simulink model "HybridPowertrain_TestBench_Final"  (R2017a)
settings: Solver=ode1  StartTime=0.0  StopTime=1400  FixedStep=0.01  RelTol=1e-3  EnableMultiTasking=on
undefined symbols (not defined in the file): AccActPos, air, Atm_temp, bms_inletair_temp, BMS_IstStrom, bms_maxchargecurrent, bms_maxdischargecurrent, BMS_Notfallkuehlung, BMS_SOC, BrkPdlPos, cal, Cells, Chg, D1_Commanded_Torque, D1_DC_Bus_Voltage, D2_Motor_Speed, D2_Torque_Feedback, DriverControls, EcoCAR3_Lib, Em, EngActStdyStTorq, Engine, EngSpd, env, ESS, fd, g, gb, Gearbox, GearBox, gps_lat, gps_long, Grade, I_loss, IMG, InstFuelConsmpRate, KeyPosition, lib_ESS_plant_V1_2, Loss, max_vehicle_rad_air_flow, mot, mph2kph, mph2ms, NeutralGear, ParkGear, PPEI_Engine_General_Status_2__ThrPos, PTEI_Engine_Torque_Status__EngActStdyStTorq, R_0, R_1, Ratio, RegenBrkDisable, rho, SampleTime, ShiftLeverPosition, SOC_bp, SOC_init, Spd, Speed, SW_CS_ON, SW_Engine_ON ... (+15)
libraries: simulink x39, fl_lib x13, nesl_utility x8, Utility x1, EC2_libraries x1
(part 5 of 5)

== system HybridPowertrain_TestBench_Final/IMG/Soft MCU/Torque Calculation/max torque /Divide by zero ==
  In1 : Inport
  Compare To Constant : simulink/Logic and Bit Operations/Compare To Constant  relop=<=  const=3.0  OutDataTypeStr=boolean
  Constant1 : Constant
  Switch2 : Switch  Criteria=u2 > Threshold
  Out1 : Outport
  wires:
  Constant1/1 -> Switch2/1
  Compare To Constant/1 -> Switch2/2
  In1/1 -> Switch2/3, Compare To Constant/1
  Switch2/1 -> Out1/1

== system HybridPowertrain_TestBench_Final/IMG/Soft MCU/Torque Calculation/max torque /Heat index ==
  note: Heat index calculation
  cont torque : Inport
  torque : Inport  Port=2
  Abs : Abs  SaturateOnIntegerOverflow=on
  Divide : Subsystem  mask(Divide){}
      mask Display: disp('Divide')
  Heat Energy Factor : Integrator  InitialCondition=-0.3  LimitOutput=on  UpperSaturationLimit=1  LowerSaturationLimit=-0.3
  Heating Constant : Gain  Gain=0.3/mot.plant.init.t_max_trq  SaturateOnIntegerOverflow=on  OutDataTypeStr=Inherit: Same as input  ParamDataTypeStr=Inherit: Same as input
  Saturation : Saturate  UpperLimit=1  LowerLimit=0
  Sum : Sum  Inputs=+-  SaturateOnIntegerOverflow=on  InputSameDT=on  OutDataTypeStr=Inherit: Same as first input
  motor inertia (Nms^2\rad)5 : Constant
  Heat index : Outport
  wires:
  cont torque/1 -> Divide/2(denominator)
  Abs/1 -> Sum/1
  Saturation/1 -> Heat index/1
  motor inertia (Nms^2\rad)5/1 -> Sum/2
  Divide/1(quotient) -> Abs/1
  Sum/1 -> Heating Constant/1
  Heating Constant/1 -> Heat Energy Factor/1
  Heat Energy Factor/1 -> Saturation/1
  torque/1 -> Divide/1(numerator)

== system HybridPowertrain_TestBench_Final/Transmission/Transmission Plant/Gearbox/Speed Calculation/P//N ==
  torque input : Inport
  Inertia Input : Inport  Port=2
  gear : Inport  Port=3
  inital speed : Inport  Port=4
  (0,inf) : Saturate  UpperLimit=1100  LowerLimit=0
  Add : Sum
  Bus Selector : BusSelector  Commented=on  OutputSignals=drv_BPP_req_[%]
  Compare To Constant : simulink/Logic and Bit Operations/Compare To Constant  Commented=on  relop=<=  const=1  OutDataTypeStr=boolean
  Compare To Constant1 : simulink/Logic and Bit Operations/Compare To Constant  Commented=on  relop=>  const=2  OutDataTypeStr=boolean
  Compare To Constant2 : simulink/Logic and Bit Operations/Compare To Constant  Commented=on  relop=<=  const=1000  OutDataTypeStr=boolean
  Fcn2 : Fcn  Expr=u==0
  From10 : From  Commented=on  GotoTag=Driver_Request  TagVisibility=global
  Inertias : Constant  Value=Gearbox.InputShaftInertia
  Integrator : Integrator  ExternalReset=rising  InitialConditionSource=external
  Logical Operator : Logic  Commented=on  Inputs=3  AllPortsSameDT=off  OutDataTypeStr=boolean
  Logical Operator1 : Logic  Operator=OR  AllPortsSameDT=off  OutDataTypeStr=boolean
  Memory : Memory
  Subsystem2 : Subsystem
      mask Display: disp('divider')
  Sum : Sum  Inputs=-+|  SaturateOnIntegerOverflow=on  InputSameDT=on  OutDataTypeStr=Inherit: Same as first input
  Switch : Switch  Commented=on  Criteria=u2 > Threshold
  input shaft free wheeling losses : Subsystem
  speed : Outport
  decel : Outport  Port=2
  wires:
  Inertia Input/1 -> Add/1
  Fcn2/1 -> Logical Operator1/2
  Subsystem2/1(Out1) -> decel/1, Integrator/1
  Memory/1 -> Integrator/3
  (0,inf)/1 -> speed/1
  torque input/1 -> Sum/2
  Sum/1 -> Subsystem2/1(In1)
  input shaft free wheeling losses/1(input shaft decel) -> Sum/1
  Integrator/1 -> input shaft free wheeling losses/1(input shaft speed), Switch/1, (0,inf)/1
  gear/1 -> Fcn2/1, Compare To Constant/1
  Compare To Constant/1 -> Logical Operator/2
  Logical Operator/1 -> Logical Operator1/1, Switch/2
  From10/1 -> Bus Selector/1
  Bus Selector/1 -> Compare To Constant1/1  "<drv_BPP_req_[%]>"
  Compare To Constant1/1 -> Logical Operator/1
  Compare To Constant2/1 -> Logical Operator/3
  inital speed/1 -> Compare To Constant2/1, Memory/1
  Logical Operator1/1 -> Integrator/2
  Add/1 -> Subsystem2/2(In2)
  Inertias/1 -> Add/2

== system HybridPowertrain_TestBench_Final/Transmission/Transmission Plant/Gearbox/Speed Calculation/R//D ==
  spd in : Inport
  gear number : Inport  Port=2
  speed1 : Inport  Port=3
  Bus Selector : BusSelector  OutputSignals=drv_BPP_req_[%]
  Compare To Constant : simulink/Logic and Bit Operations/Compare To Constant  relop=<=  const=1  OutDataTypeStr=boolean
  Compare To Constant1 : simulink/Logic and Bit Operations/Compare To Constant  relop=>  const=0.4  OutDataTypeStr=boolean
  Compare To Constant2 : simulink/Logic and Bit Operations/Compare To Constant  relop=<=  const=1000  OutDataTypeStr=boolean
  Constant5 : Constant
  Constant6 : Constant  Value=gb.plant.init.shift_time
  Integrator : Integrator  ExternalReset=rising
  Logical Operator : Logic  Inputs=3  AllPortsSameDT=off  OutDataTypeStr=boolean
  Relational Operator4 : RelationalOperator  Operator=~=  RndMeth=Nearest  InputSameDT=on
  Relational Operator5 : RelationalOperator  Operator=<=  RndMeth=Nearest  InputSameDT=on
  S-R Flip-Flop : Subsystem  mask(SRFlipFlop){initial_condition=0}
      mask prompts: initial_condition "Initial condition:"
      mask help: S-R Flip Flop Block
  Switch : Switch  Threshold=0.5  SaturateOnIntegerOverflow=on  InputSameDT=on
  Switch1 : Switch  Criteria=u2 > Threshold
  Transfer Fcn : TransferFcn  Denominator=[.2 1]
  Unit Delay7 : Memory
  term2 : Terminator
  spd in filtered : Outport
  wires:
  spd in/1 -> Transfer Fcn/1, Switch/3, Switch1/3, Compare To Constant2/1
  Relational Operator5/1 -> S-R Flip-Flop/2(R)
  S-R Flip-Flop/1(Q) -> Switch/2
  Integrator/1 -> Relational Operator5/2
  Relational Operator4/1 -> S-R Flip-Flop/1(S), Integrator/2
  Unit Delay7/1 -> Relational Operator4/2
  S-R Flip-Flop/2(!Q) -> term2/1
  Constant6/1 -> Relational Operator5/1
  Constant5/1 -> Integrator/1
  gear number/1 -> Compare To Constant/1, Unit Delay7/1, Relational Operator4/1
  [Driver_Request2] -> Bus Selector/1
  Bus Selector/1 -> Compare To Constant1/1  "<drv_BPP_req_[%]>"
  Compare To Constant1/1 -> Logical Operator/1
  Compare To Constant/1 -> Logical Operator/2
  Logical Operator/1 -> Switch1/2
  Compare To Constant2/1 -> Logical Operator/3
  Switch1/1 -> spd in filtered/1
  speed1/1 -> Switch1/1
  Transfer Fcn/1 -> Switch/1

== system HybridPowertrain_TestBench_Final/Transmission/Transmission Plant/Gearbox/Subsystem1/Blending (state dependent) ==
  Input : Inport
  Control (state) : Inport  Port=2
  Linear spline : Fcn  Expr=(u<xl)*yl + (xl<=u)*(u<xc)*((yc-yl)*(u-xl)/(xc-xl)+yl) + (xc<=u)*(u<xr)*((yc-yr)*(u-xr)/(xc-xr)+yr) + (xr<=u)*yr
  Product2 : Product  SaturateOnIntegerOverflow=on  InputSameDT=on  OutDataTypeStr=Inherit: Same as first input
  Output : Outport
  wires:
  Control (state)/1 -> Linear spline/1
  Product2/1 -> Output/1
  Linear spline/1 -> Product2/2
  Input/1 -> Product2/1

== system HybridPowertrain_TestBench_Final/Transmission/Transmission Plant/Gearbox/Torque calculation/Blending (state dependent) ==
  Input : Inport
  Control (state) : Inport  Port=2
  Linear spline : Fcn  Expr=(u<xl)*yl + (xl<=u)*(u<xc)*((yc-yl)*(u-xl)/(xc-xl)+yl) + (xc<=u)*(u<xr)*((yc-yr)*(u-xr)/(xc-xr)+yr) + (xr<=u)*yr
  Product2 : Product  SaturateOnIntegerOverflow=on  InputSameDT=on  OutDataTypeStr=Inherit: Same as first input
  Output : Outport
  wires:
  Control (state)/1 -> Linear spline/1
  Product2/1 -> Output/1
  Linear spline/1 -> Product2/2
  Input/1 -> Product2/1

== system HybridPowertrain_TestBench_Final/ESS/Soft BMS/Limits/Average Current/60 sec rolling average1/1sec trigger ==
  0 : Constant  Value=0
  Compare To Constant : simulink/Logic and Bit Operations/Compare To Constant  relop=<=  const=3.0  OutDataTypeStr=boolean
  Data Type Conversion : DataTypeConversion
  Sum2 : Sum  Inputs=|++
  Switch : Switch  Threshold=0.5
  accumulate2 : Memory  InheritSampleTime=on
  tloop : Constant  Value=tloop
  Trigger : Outport
  wires:
  Data Type Conversion/1 -> Trigger/1, Switch/2
  0/1 -> Switch/1
  Compare To Constant/1 -> Data Type Conversion/1
  Switch/1 -> accumulate2/1
  Sum2/1 -> Switch/3, Compare To Constant/1
  accumulate2/1 -> Sum2/2
  tloop/1 -> Sum2/1

== system HybridPowertrain_TestBench_Final/ESS/Soft BMS/Limits/Average Current/60 sec rolling average1/60 sec average ==
  1sec : Inport
  Enable : EnablePort
  60 second : Delay  DelayLength=60  InputProcessing=Inherited  SampleTime=tloop
  Gain2 : Gain  Gain=1/60
  Sum2 : Sum  Inputs=++-
  accumulate2 : Memory  InheritSampleTime=on
  Average : Outport
  wires:
  1sec/1 -> Sum2/2, 60 second/1
  Gain2/1 -> Average/1
  accumulate2/1 -> Sum2/1
  60 second/1 -> Sum2/3
  Sum2/1 -> Gain2/1, accumulate2/1

== system HybridPowertrain_TestBench_Final/ESS/Soft BMS/Limits/Average Current/60 sec rolling average2/1sec trigger ==
  0 : Constant  Value=0
  Compare To Constant : simulink/Logic and Bit Operations/Compare To Constant  relop=<=  const=3.0  OutDataTypeStr=boolean
  Data Type Conversion : DataTypeConversion
  Sum2 : Sum  Inputs=|++
  Switch : Switch  Threshold=0.5
  accumulate2 : Memory  InheritSampleTime=on
  tloop : Constant  Value=tloop
  Trigger : Outport
  wires:
  Data Type Conversion/1 -> Trigger/1, Switch/2
  0/1 -> Switch/1
  Compare To Constant/1 -> Data Type Conversion/1
  Switch/1 -> accumulate2/1
  Sum2/1 -> Switch/3, Compare To Constant/1
  accumulate2/1 -> Sum2/2
  tloop/1 -> Sum2/1

== system HybridPowertrain_TestBench_Final/ESS/Soft BMS/Limits/Average Current/60 sec rolling average2/60 sec average ==
  1sec : Inport
  Enable : EnablePort
  60 second : Delay  DelayLength=60  InputProcessing=Inherited  SampleTime=tloop
  Gain2 : Gain  Gain=1/60
  Sum2 : Sum  Inputs=++-
  accumulate2 : Memory  InheritSampleTime=on
  Average : Outport
  wires:
  1sec/1 -> Sum2/2, 60 second/1
  Gain2/1 -> Average/1
  accumulate2/1 -> Sum2/1
  60 second/1 -> Sum2/3
  Sum2/1 -> Gain2/1, accumulate2/1

== system HybridPowertrain_TestBench_Final/IMG/Soft MCU/Torque Calculation/max torque /Heat index/Divide ==
  note: Take care of
      | division by 0
  numerator : Inport
  denominator : Inport  Port=2
  Fcn : Fcn  Expr=u[1] / ( u[2] + eps*(u[2]==0) )
  Mux : Mux  Inputs=2
  quotient : Outport
  wires:
  denominator/1 -> Mux/2
  Fcn/1 -> quotient/1
  numerator/1 -> Mux/1
  Mux/1 -> Fcn/1

== system HybridPowertrain_TestBench_Final/Transmission/Transmission Plant/Gearbox/Speed Calculation/P//N/Subsystem2 ==
  In1 : Inport
  In2 : Inport  Port=2
  Fcn : Fcn  Expr=u[1]/(u[2]+eps)*(u[2]!=0)
  Mux : Mux  Inputs=2
  Out1 : Outport
  wires:
  Mux/1 -> Fcn/1
  In1/1 -> Mux/1
  Fcn/1 -> Out1/1
  In2/1 -> Mux/2

== system HybridPowertrain_TestBench_Final/Transmission/Transmission Plant/Gearbox/Speed Calculation/P//N/input shaft free wheeling losses ==
  input shaft speed : Inport
  Constant1 : Constant  Value=0
  Fcn1 : Fcn  Expr=u==0
  Gain1 : Gain  Gain=0.15  SaturateOnIntegerOverflow=on  OutDataTypeStr=Inherit: Same as input  ParamDataTypeStr=Inherit: Same as input
  Switch2 : Switch  Threshold=0.5  SaturateOnIntegerOverflow=on  InputSameDT=on
  input shaft decel : Outport
  wires:
  input shaft speed/1 -> Switch2/3, Fcn1/1
  Fcn1/1 -> Switch2/2
  Gain1/1 -> input shaft decel/1
  Switch2/1 -> Gain1/1
  Constant1/1 -> Switch2/1

== system HybridPowertrain_TestBench_Final/Transmission/Transmission Plant/Gearbox/Speed Calculation/R//D/S-R Flip-Flop ==
  S : Inport
  R : Inport  Port=2
  Demux : Demux  Outputs=2
  Logic : CombinatorialLogic  TruthTable=[0 1;0 1;1 0;0 1;1 0;0 1;1 0;1 0]
  Memory : Memory  X0=initial_condition  InheritSampleTime=on
  Mux : Mux  Inputs=3
  Q : Outport  InitialOutput=0
  !Q : Outport  Port=2  InitialOutput=1
  wires:
  R/1 -> Mux/3
  S/1 -> Mux/2
  Memory/1 -> Mux/1
  Demux/1 -> Memory/1, Q/1
  Demux/2 -> !Q/1
  Logic/1 -> Demux/1
  Mux/1 -> Logic/1

== stateflow chart HybridPowertrain_TestBench_Final/ESS/Soft BMS/RollingAliveCnt1/Rolling Alive Counter ==
  state RollingAliveCounter
    state Count1
      en: RollingAliveCnt = 0;
    state Count2
      en: RollingAliveCnt = 1;
    state Count3
      en: RollingAliveCnt = 2;
    state Count4
      en: RollingAliveCnt = 3;
    (default) -> Count1
    Count4 -> Count1 : after(0.01,sec)
    Count1 -> Count2 : after(0.01,sec)
    Count2 -> Count3 : after(0.01,sec)
    Count3 -> Count4 : after(0.01,sec)
  data: RollingAliveCnt output int8 =0

== stateflow chart HybridPowertrain_TestBench_Final/ESS/Soft BMS/State Machine1/Startup_Shutdown_EPO_Sequence ==
  state BCM_ON
    state Default_Error_State
      en: BMS_Init_abgeschlossen=1;
      BMS_IstModus=5;
    state Standby
      en: BMS_Init_abgeschlossen=1;
      BMS_IstModus=0;
    state Normal_Driving
      en: NHM_BMS_Car_WakeUp=1;
      BMS_IstModus=1;
      BMS_Init_abgeschlossen=1;
      during: timer++;
    state Charging
      en:BMS_IstModus=4;
      BMS_Init_abgeschlossen =1;
      during: timer++;
    (default) -> Default_Error_State : [T_15&&T_30]
    Charging -> Default_Error_State [order 1] : [!T_30C]
    Normal_Driving -> Default_Error_State [order 1] : [!T_30C]
    (junction 134) -> Default_Error_State [order 2] : after(15, sec)[!T_30C]
    Default_Error_State -> Standby : [MO_BMS_Sollmodus==0&&...
        | Diag_Rq_Fktnl_Data_OBD==1]
        | %ErrorClear
    (junction 134) -> Standby [order 1] : [T_30C]
    Standby -> (junction 134) [order 3] : [!T_30C]
    Standby -> Charging [order 1] : [T_30C&&MO_BMS_Sollmodus==4]
        | %Standby>Charging
    Standby -> Normal_Driving [order 2] : [T_30C&&MO_BMS_Sollmodus==1]
        | {timer=0;}
        | %Standby>NormalDriving
    Normal_Driving -> Standby [order 2] : [T_30C&&MO_BMS_Sollmodus==0]
        | %NormalDriving>Standby
    Charging -> Standby [order 2] : [T_30C&&MO_BMS_Sollmodus==0]
        | %Charging>Standby
    Normal_Driving -> Charging [order 3] : [T_30C&&MO_BMS_Sollmodus==4] %NormalDriving>Charging
    Charging -> Normal_Driving [order 3] : [T_30C&&MO_BMS_Sollmodus==1] %Charging>NormalDriving
  state BCM_OFF
    state Prepare_to_Sleep
      en: NMH_BMS_Start_2=0;
      BMS_IstModus=5;
    state Ready_to_Sleep
      en: NMH_BMS_Normal_Mode_2=0;
      BMS_SleepInd=1;
      BMS_IstModus=5;
    state Bus_Sleep
      en: NMH_BMS_Start_1=0;
      BMS_SleepInd=1;
      BMS_IstModus=5;
    (default) -> Prepare_to_Sleep
    Prepare_to_Sleep -> Ready_to_Sleep : [timer>=0.05/tloop]
    Ready_to_Sleep -> Bus_Sleep : [timer>=0.05/tloop]
  note: !(veh_wake||chga_wake) || ...
      | !hsc_bcm_enable && !bcm_mainc_stat && bcm_cpwr_cmd]
  state EPO1
    BMS_Fehler_HS_offen=1;
    BMS_Fehler_HS_verschweisst =1;
    BMS_Fehler_HVBatt_Abschaltung=1;
    BMS_Fehler_HVBatt_Abschaltung_Anf=1;
    BMS_IstModus=5;
  state EPO
    BMS_Fehler_Notabschaltung_Crash=1;
    BMS_Fehler_Notabschaltung_Pilot=1;
    BMS_Fehler_Pilot=1;
    BMS_IstModus=5;
  (default) -> BCM_OFF
  BCM_OFF -> BCM_ON : [T_15&&T_30]
  BCM_ON -> BCM_OFF [order 1] : [T_15==0&&T_30==0]
  BCM_ON -> EPO1 [order 2] : [BattError]
  EPO1 -> BCM_OFF : [T_15==0&&T_30==0]
  EPO -> BCM_OFF : [T_15==0&&T_30==0]
  BCM_ON -> EPO [order 3] : after(2,sec)[CriticalBattError||MO_Fehler_Notentladung_Anf]
  data: on_plug input boolean; timer local double; tloop parameter double; T_15 input double; T_30 input double; MO_BMS_Sollmodus input double; T_30C input double; BMS_Init_abgeschlossen output double; BMS_IstModus output double; BMS_Fehler_Pilot output double; NMH_Normal_Mode_1 output double; BMS_Fehler_HS_offen output double; BMS_Fehler_HS_verschweisst output double; NMH_BMS_Start_2 output double; NMH_BMS_Start_1 output double; BMS_Fehler_Notabschaltung_Crash output double; BMS_Fehler_Notabschaltung_Pilot output double; NHM_BMS_Car_WakeUp output double; BMS_SleepInd output double; NMH_BMS_Normal_Mode_2 output double; MO_Fehler_Notentladung_Anf input double; Diag_Rq_Fktnl_Data_OBD input boolean; BattError input boolean; CriticalBattError input boolean; BMS_Fehler_HVBatt_Abschaltung output double; BMS_Fehler_HVBatt_Abschaltung_Anf output double

== stateflow chart HybridPowertrain_TestBench_Final/ICE Simple/Engine Plant Modified/Core Engine/Crank Process ==
  state Starter_Crank
    du:
    EngActTrq = function(EngSpd_RPM);
  state Eng_Off
    du:
    EngActTrq = 0;
  state Eng_Combustion
    du:
    EngActTrq = 100;
  state CrankTrq = function(EngSpd) [function]
  state Eng_Run
    du:
    EngActTrq = EngBrkTrq;
  (default) -> Eng_Off
  Eng_Off -> Starter_Crank : [EngCrankCmd]
  Starter_Crank -> Eng_Off [order 2] : [!EngCrankCmd]
  Eng_Run -> Eng_Off : [AvlblFuel <= 0.01|| EngShutdown == 1]
  Starter_Crank -> Eng_Combustion [order 1] : [AvlblFuel >= 0.1]
  Eng_Combustion -> Eng_Run : [EngRunAtv]
  data: CrankTrq function_output; EngSpd function_input; EngRunAtv input boolean; AvlblFuel input double; EngActTrq output double; EngCrankCmd input boolean; EngBrkTrq input double; EngSpd_RPM input double; EngShutdown input boolean

== stateflow chart HybridPowertrain_TestBench_Final/ICE Simple/Soft ECM/ECM_RollingAliveCnt/Rolling Alive Counter ==
  state RollingAliveCounter
    state Count1
      en: RollingAliveCnt = 0;
    state Count2
      en: RollingAliveCnt = 1;
    state Count3
      en: RollingAliveCnt = 2;
    state Count4
      en: RollingAliveCnt = 3;
    (default) -> Count1
    Count4 -> Count1 : after(0.01,sec)
    Count1 -> Count2 : after(0.01,sec)
    Count2 -> Count3 : after(0.01,sec)
    Count3 -> Count4 : after(0.01,sec)
  data: RollingAliveCnt output int8 =0

== stateflow chart HybridPowertrain_TestBench_Final/ICE Simple/Soft ECM/Logic ==
  state Eng_Off
    en:
    EngRunAtv = 0;
    EngCrankCmd = 0;
    FuelPumpEnable = 0;
    du:
    ThrottleCmd = APP2TP(EngSpd_RPM,drvAPP,ShftLvrPos);
  state Eng_Crank
    en:
    EngCrankCmd = 1;
    FuelPumpEnable = 1;
    EngShutdown = 0;
  state Eng_On
    en:
    EngRunAtv = 1;
    EngCrankCmd = 0;
    du:
    ThrottleCmd = APP2TP(EngSpd_RPM,drvAPP,ShftLvrPos);
  state TP = APP2TP(EngSpd,APP,Shifter) [function]
  (default) -> Eng_Off
  Eng_Off -> Eng_Crank : [SysPwrMd == 3]
  Eng_Crank -> Eng_Off [order 2] : [SysPwrMd < 3]
  Eng_Crank -> Eng_On [order 1] : [EngSpd_RPM >= 580]
  Eng_On -> Eng_Off : [SysPwrMd < 2 || EngSpd_RPM < 500]
      | {EngShutdown = 1; }
  data: EngSpd function_input; TP function_output; APP function_input; Shifter function_input; drvAPP input; ThrottleCmd output double; EngCrankCmd output boolean; SysPwrMd input int8; ShftLvrPos input int8; EngSpd_RPM input double; VehSpdAvgDrvn input double; EngRunAtv output boolean; FuelPumpEnable output double; EngShutdown output boolean

== stateflow chart HybridPowertrain_TestBench_Final/IMG/Soft MCU/MCU_CAN_rolling/Rolling Alive Counter1 ==
  state RollingAliveCounter
    state Count1
      en: RollingAliveCnt=0;
    state Count2
      en: RollingAliveCnt=1;
    state Count3
      en: RollingAliveCnt=2;
    state Count4
      en: RollingAliveCnt=3;
    (default) -> Count1
    Count4 -> Count1 : after(0.01,sec)
    Count1 -> Count2 : after(0.01,sec)
    Count2 -> Count3 : after(0.01,sec)
    Count3 -> Count4 : after(0.01,sec)
  data: RollingAliveCnt output double

== stateflow chart HybridPowertrain_TestBench_Final/Transmission/Soft TCM/6L45 Logic ==
  settings: sampleTime=0.04
  state Torque_Converter_Control [parallel]
    du:
    du:[lockup_thrsh]=calc_lockup(Gear_D, drvAPP);
    du:[unlock_thrsh]=calc_unlock(Gear_D, drvAPP);
    settings: executionOrder=1
    state lockup_th = calc_lockup(Gear, APP) [function]
    note: Lever Position:
        | 1 P
        | 2 R
        | 3 N
        | 4 D
        |
        | 1 clutch lock-up
        | 0 clutch unlock
    state Lock
      en:
      LockupCmd = 1;
    state Unlock
      en:
      LockupCmd = 0;
    state unlock_th = calc_unlock(Gear,APP) [function]
    (default) -> Unlock
    Unlock -> Lock : [(Gear_D >= 4 || drvBPP > 0) && VehicleSpeed > 20]
    Lock -> Unlock : [VehicleSpeed < 20 || drvBPP == 0 && drvAPP > 5 && Gear_D <= 3]
  state Gearbox_Control [parallel]
    settings: executionOrder=2
    state Shifter_Actuator [parallel]
      settings: executionOrder=1
      state Shifter_D
        du:
        TransEstGear = Gear_D;
      state Shifter_R
        en:
        TransEstGear = 14;
      state Shifter_N
        en:
        TransEstGear = 13;
      state Shifter_P
        en:
        TransEstGear = 15;
      (default) -> Shifter_P
      Shifter_D -> Shifter_N : [ShftLvrPos <= 3]
      Shifter_N -> Shifter_R [order 2] : [ShftLvrPos <= 2]
      Shifter_R -> Shifter_P [order 2] : [ShftLvrPos <= 1]
      Shifter_N -> Shifter_D [order 1] : [ShftLvrPos >= 4]
      Shifter_R -> Shifter_N [order 1] : [ShftLvrPos >= 3]
      Shifter_P -> Shifter_R : [ShftLvrPos >= 2]
    state Shift_Schedule [parallel]
      settings: executionOrder=2
      state Gear_State_D [parallel]
        settings: executionOrder=1
        state Gear_4th
          entry:
          Gear_D = 4;
        state Gear_3rd
          entry:
          Gear_D = 3;
        state Gear_6th
          entry:
          Gear_D = 6;
        state Gear_7th
          entry:
          Gear_D = 7;
        state Gear_8th
          entry:
          Gear_D = 8;
        state Gear_1st
          entry:
          Gear_D = 1;
        state Gear_5th
          entry:
          Gear_D = 5;
        state Gear_2nd
          entry:
          Gear_D  = 2;
        (default) -> Gear_1st
        Gear_2nd -> Gear_3rd [order 1] : UP
        Gear_7th -> Gear_8th [order 1] : UP
        Gear_4th -> Gear_5th [order 1] : UP
        Gear_5th -> Gear_6th [order 1] : UP
        Gear_6th -> Gear_7th [order 1] : UP
        Gear_3rd -> Gear_4th [order 1] : UP
        Gear_1st -> Gear_2nd : UP
        Gear_3rd -> Gear_2nd [order 2] : DOWN
        Gear_4th -> Gear_3rd [order 2] : DOWN
        Gear_2nd -> Gear_1st [order 2] : DOWN
        Gear_5th -> Gear_4th [order 2] : DOWN
        Gear_6th -> Gear_5th [order 2] : DOWN
        Gear_7th -> Gear_6th [order 2] : DOWN
        Gear_8th -> Gear_7th : DOWN
      state Gear_Transient_D [parallel]
        du:[up_thrsh]=calc_up(Gear_D, drvAPP);
        du:[down_thrsh]=calc_down(Gear_D, drvAPP);
        settings: executionOrder=2
        state steady_state
        state upshifting
        state downshifting
        (default) -> steady_state
        steady_state -> upshifting [order 1] : [VehicleSpeed > up_thrsh && Gear_D < 8]
        steady_state -> downshifting [order 2] : [VehicleSpeed < down_thrsh && Gear_D > 1]
        downshifting -> steady_state [order 1] : after(0.1,sec)
            | [VehicleSpeed <= down_thrsh]
            | {Gear_State_D.DOWN;}
        downshifting -> steady_state [order 2] : [VehicleSpeed > down_thrsh]
        upshifting -> steady_state [order 1] : after(0.1,sec)
            | [VehicleSpeed >= up_thrsh]
            | {Gear_State_D.UP;}
        upshifting -> steady_state [order 2] : [VehicleSpeed < up_thrsh]
      state PlotShiftSchedule [function]
      state up_th = calc_up(Gear, APP) [function]
      state down_th = calc_down(Gear, APP) [function]
  data: Gear function_input; APP function_input; lockup_th function_output; Gear function_input; APP function_input; unlock_th function_output; Gear function_input; APP function_input; up_th function_output; Gear function_input; APP function_input; down_th function_output; tc_lockup_thrsh input double; Gear_D local int8 =1; drvAPP input double [0..100]; VehicleSpeed input double; TransEstGear output int8; down_thrsh local double =0; up_thrsh local double =0; LockupCmd output boolean; tc_spd_in input double; tc_spd_out input double; drvBPP input double; ShftLvrPos input int8; lockup_thrsh local double; unlock_thrsh local double
  events: DOWN local EITHER_EDGE_EVENT; UP local EITHER_EDGE_EVENT

== stateflow chart HybridPowertrain_TestBench_Final/ESS/Soft BMS/BMS_HYB_1/BMS_HYB_02_BZ/Rolling Alive Counter ==
  state RollingAliveCounter
    state Count1
      en: RollingAliveCnt = 0;
    state Count2
      en: RollingAliveCnt = 1;
    state Count3
      en: RollingAliveCnt = 2;
    state Count4
      en: RollingAliveCnt = 3;
    (default) -> Count1
    Count4 -> Count1 : after(0.01,sec)
    Count1 -> Count2 : after(0.01,sec)
    Count2 -> Count3 : after(0.01,sec)
    Count3 -> Count4 : after(0.01,sec)
  data: RollingAliveCnt output int8 =0
